simulink model "mba_model_linear"  (R2016a)
settings: Solver=VariableStepAuto  StartTime=0.0  StopTime=.1  RelTol=1e-5
undefined symbols (not defined in the file or in its folder): k, u0, x0
settings Model: Creator=manuel  LastModifiedBy=manuel

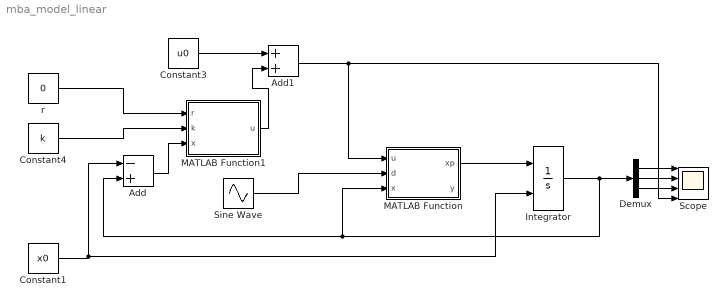
== system mba_model_linear ==
  Add : Sum  Inputs=-+
  Add1 : Sum
  Constant1 : Constant  Value=x0
  Constant3 : Constant  Value=u0
  Constant4 : Constant  Value=k
  Demux : Demux  Outputs=3
  Integrator : Integrator  InitialConditionSource=external  InitialCondition=[1.5e-3;0;0.4805]  LimitOutput=on  UpperSaturationLimit=[3e-3;inf;5]  LowerSaturationLimit=[.8e-3;-inf;-0.5]
  MATLAB Function : MATLAB Function  TreatAsAtomicUnit=on
  MATLAB Function1 : MATLAB Function  TreatAsAtomicUnit=on
  Scope : Scope  NumInputPorts=4
  Sine Wave : Sin  Amplitude=0.4  Bias=0.2  Frequency=1000  SampleTime=0
  r : Constant  Value=0
  wires:
  MATLAB Function/1(xp) -> Integrator/1
  MATLAB Function1/1(u) -> Add1/2
  Integrator/1 -> MATLAB Function/3(x), Add/2, Demux/1
  r/1 -> MATLAB Function1/1(r)
  Sine Wave/1 -> MATLAB Function/2(d)
  Demux/1 -> Scope/1
  Demux/2 -> Scope/2
  Demux/3 -> Scope/3
  Constant1/1 -> Add/1, Integrator/2
  Add/1 -> MATLAB Function1/3(x)
  Constant3/1 -> Add1/1
  Add1/1 -> Scope/4, MATLAB Function/1(u)
  Constant4/1 -> MATLAB Function1/2(k)

== matlab function mba_model_linear/MATLAB Function1 ==
  data: r input; k input; x input; u output
function u = controller(r,k,x)
%#codegen
u = r-k'*x;

if(u < -24)
   u = -24;
elseif(u > 24)
   u = 24;
end

== matlab function mba_model_linear/MATLAB Function ==
  data: u input; d input; x input; xp output; y output
function [xp,y] = mba_ss(u,d,x)
%#codegen

m = .1;
[F,Vfem,R,L] = get_electromagnet_parameters(x(1),x(2),x(3));

xp = [  x(2);
        (d+F+(9.8*m))/m;
        ((u-Vfem-(x(3)*R))/L)];

C = [1 0 0;
     0 1 0];

y = C*x;
